simulink library "Bit_Multiplexers_Lib"  (R2023a)
settings: Solver=ode45  StartTime=0.0  StopTime=10.0  RelTol=1e-3  EnableMultiTasking=on
settings Model: Creator=uzivatel  LastModifiedBy=Jozko Mrkvicka
settings SolverCC: AlgebraicLoopSolver=TrustRegion
settings DataIOCC: LimitDataPoints=on  SaveFormat=Array  ReturnWorkspaceOutputs=off
settings OptimizationCC: LifeSpan=inf
settings DebuggingCC: UnderspecifiedInitializationDetection=Classic  MergeDetectMultiDrivingBlocksExec=none  SolverPrmCheckMsg=warning  UnconnectedInputMsg=warning  UnconnectedOutputMsg=warning  UnconnectedLineMsg=warning  StateNameClashWarn=warning  SFUnexpectedBacktrackingDiag=warning  SFNoUnconditionalDefaultTransitionDiag=warning  ArithmeticOperatorsInVariantConditions=warning
settings HardwareCC: ProdBitPerPointer=32  ProdBitPerSizeT=32  ProdBitPerPtrDiffT=32  ProdLargestAtomicFloat=None  ProdIntDivRoundTo=Undefined  ProdEndianess=Unspecified  ProdWordSize=32  ProdHWDeviceType=32-bit Generic
settings ModelReferenceCC: EnableRefExpFcnMdlSchedulingChecks=on  PropagateSignalLabelsOutOfModel=off
settings SFSimCC: SimUseLocalCustomCode=off  CustomCodeUndefinedFunction=UseInterfaceOnly
settings RTWCC: RTWUseLocalCustomCode=off
settings CodeAppCC: StateflowObjectComments=on
settings GRTTargetCC: TargetLangStandard=C89/C90 (ANSI)
settings ConfigComp: CovMetricSettings=dw  CovSaveCumulativeToWorkspaceVar=on  CovSaveSingleToWorkspaceVar=on  CovExternalEMLEnable=off

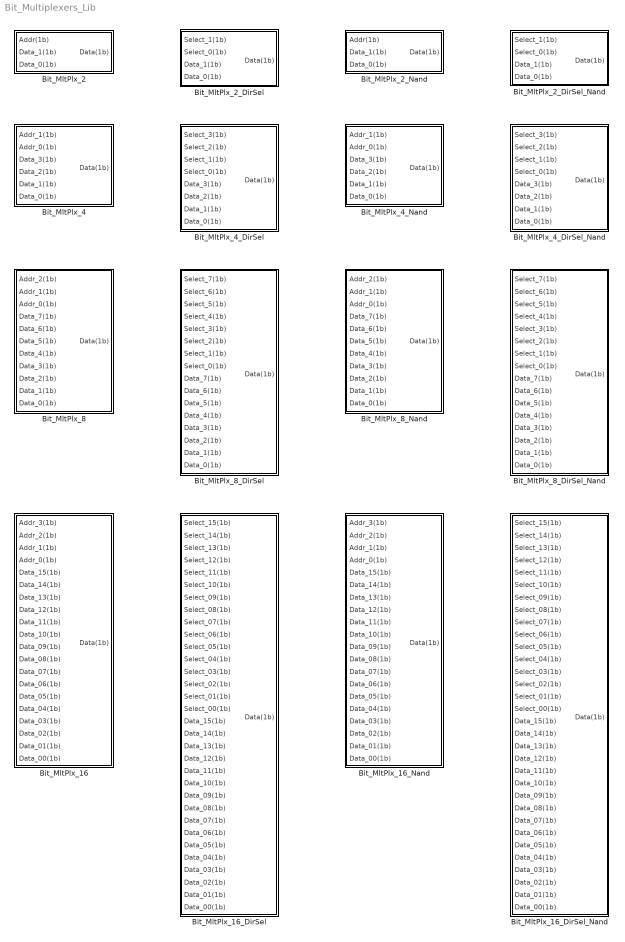
== system Bit_Multiplexers_Lib ==
  Bit_MltPlx_16 : Subsystem
  Bit_MltPlx_16_DirSel : Subsystem
  Bit_MltPlx_16_DirSel_Nand : Subsystem
  Bit_MltPlx_16_Nand : Subsystem
  Bit_MltPlx_2 : Subsystem
  Bit_MltPlx_2_DirSel : Subsystem
  Bit_MltPlx_2_DirSel_Nand : Subsystem
  Bit_MltPlx_2_Nand : Subsystem
  Bit_MltPlx_4 : Subsystem
  Bit_MltPlx_4_DirSel : Subsystem
  Bit_MltPlx_4_DirSel_Nand : Subsystem
  Bit_MltPlx_4_Nand : Subsystem
  Bit_MltPlx_8 : Subsystem
  Bit_MltPlx_8_DirSel : Subsystem
  Bit_MltPlx_8_DirSel_Nand : Subsystem
  Bit_MltPlx_8_Nand : Subsystem

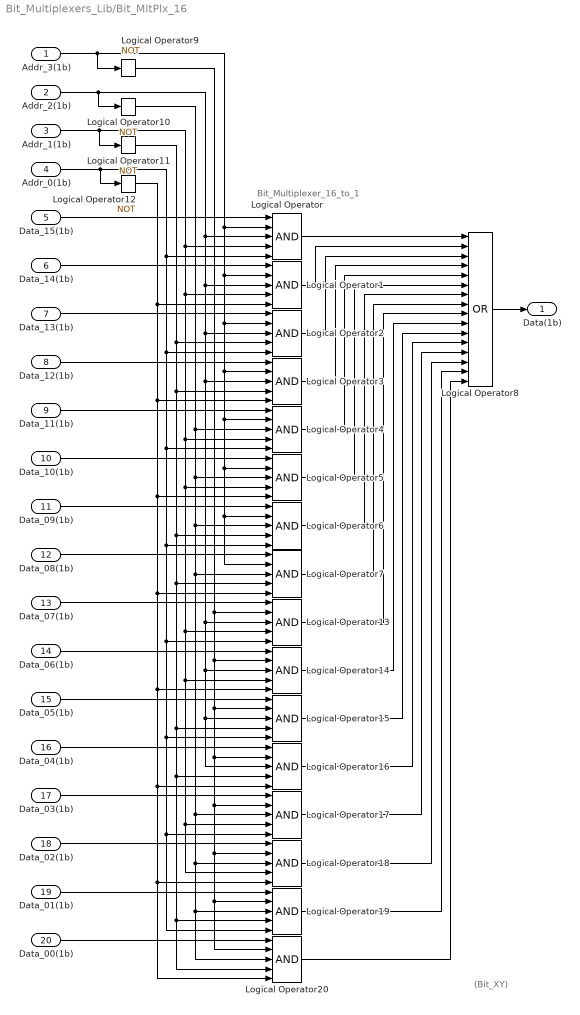
== system Bit_Multiplexers_Lib/Bit_MltPlx_16 ==
  note: (Bit_XY)
  note: Bit_Multiplexer_16_to_1
  Addr_3(1b) : Inport
  Addr_2(1b) : Inport  Port=2
  Addr_1(1b) : Inport  Port=3
  Addr_0(1b) : Inport  Port=4
  Data_15(1b) : Inport  Port=5
  Data_14(1b) : Inport  Port=6
  Data_13(1b) : Inport  Port=7
  Data_12(1b) : Inport  Port=8
  Data_11(1b) : Inport  Port=9
  Data_10(1b) : Inport  Port=10
  Data_09(1b) : Inport  Port=11
  Data_08(1b) : Inport  Port=12
  Data_07(1b) : Inport  Port=13
  Data_06(1b) : Inport  Port=14
  Data_05(1b) : Inport  Port=15
  Data_04(1b) : Inport  Port=16
  Data_03(1b) : Inport  Port=17
  Data_02(1b) : Inport  Port=18
  Data_01(1b) : Inport  Port=19
  Data_00(1b) : Inport  Port=20
  Logical Operator{,1..7,13..20} (16 alike) : Logic  Inputs=5  IconShape=distinctive  AllPortsSameDT=off  OutDataTypeStr=boolean
  Logical Operator{9..12} (4 alike) : Logic  Operator=NOT  Inputs=4  IconShape=distinctive  AllPortsSameDT=off  OutDataTypeStr=boolean
  Logical Operator8 : Logic  Operator=OR  Inputs=16  IconShape=distinctive  OutDataTypeStr=boolean
  Data(1b) : Outport
  wires:
  Logical Operator12/1 -> Logical Operator20/5, Logical Operator18/5, Logical Operator16/5, Logical Operator14/5, Logical Operator7/5, Logical Operator5/5, Logical Operator3/5, Logical Operator1/5
  Addr_0(1b)/1 -> Logical Operator19/5, Logical Operator17/5, Logical Operator15/5, Logical Operator13/5, Logical Operator6/5, Logical Operator4/5, Logical Operator2/5, Logical Operator/5, Logical Operator12/1
  Logical Operator11/1 -> Logical Operator20/4, Logical Operator19/4, Logical Operator16/4, Logical Operator15/4, Logical Operator7/4, Logical Operator6/4, Logical Operator3/4, Logical Operator2/4
  Addr_1(1b)/1 -> Logical Operator18/4, Logical Operator17/4, Logical Operator14/4, Logical Operator13/4, Logical Operator5/4, Logical Operator4/4, Logical Operator1/4, Logical Operator/4, Logical Operator11/1
  Logical Operator10/1 -> Logical Operator20/3, Logical Operator19/3, Logical Operator18/3, Logical Operator17/3, Logical Operator7/3, Logical Operator6/3, Logical Operator5/3, Logical Operator4/3
  Addr_2(1b)/1 -> Logical Operator16/3, Logical Operator15/3, Logical Operator14/3, Logical Operator13/3, Logical Operator3/3, Logical Operator2/3, Logical Operator1/3, Logical Operator/3, Logical Operator10/1
  Logical Operator9/1 -> Logical Operator20/2, Logical Operator19/2, Logical Operator18/2, Logical Operator17/2, Logical Operator16/2, Logical Operator15/2, Logical Operator14/2, Logical Operator13/2
  Addr_3(1b)/1 -> Logical Operator7/2, Logical Operator6/2, Logical Operator5/2, Logical Operator4/2, Logical Operator3/2, Logical Operator2/2, Logical Operator1/2, Logical Operator/2, Logical Operator9/1
  Data_00(1b)/1 -> Logical Operator20/1
  Data_01(1b)/1 -> Logical Operator19/1
  Data_02(1b)/1 -> Logical Operator18/1
  Data_03(1b)/1 -> Logical Operator17/1
  Data_04(1b)/1 -> Logical Operator16/1
  Data_05(1b)/1 -> Logical Operator15/1
  Data_06(1b)/1 -> Logical Operator14/1
  Data_07(1b)/1 -> Logical Operator13/1
  Logical Operator20/1 -> Logical Operator8/16
  Logical Operator19/1 -> Logical Operator8/15
  Logical Operator18/1 -> Logical Operator8/14
  Logical Operator17/1 -> Logical Operator8/13
  Logical Operator16/1 -> Logical Operator8/12
  Logical Operator15/1 -> Logical Operator8/11
  Logical Operator14/1 -> Logical Operator8/10
  Logical Operator13/1 -> Logical Operator8/9
  Logical Operator8/1 -> Data(1b)/1
  Data_15(1b)/1 -> Logical Operator/1
  Data_14(1b)/1 -> Logical Operator1/1
  Data_13(1b)/1 -> Logical Operator2/1
  Data_12(1b)/1 -> Logical Operator3/1
  Data_11(1b)/1 -> Logical Operator4/1
  Data_10(1b)/1 -> Logical Operator5/1
  Data_09(1b)/1 -> Logical Operator6/1
  Data_08(1b)/1 -> Logical Operator7/1
  Logical Operator7/1 -> Logical Operator8/8
  Logical Operator6/1 -> Logical Operator8/7
  Logical Operator5/1 -> Logical Operator8/6
  Logical Operator4/1 -> Logical Operator8/5
  Logical Operator3/1 -> Logical Operator8/4
  Logical Operator2/1 -> Logical Operator8/3
  Logical Operator1/1 -> Logical Operator8/2
  Logical Operator/1 -> Logical Operator8/1

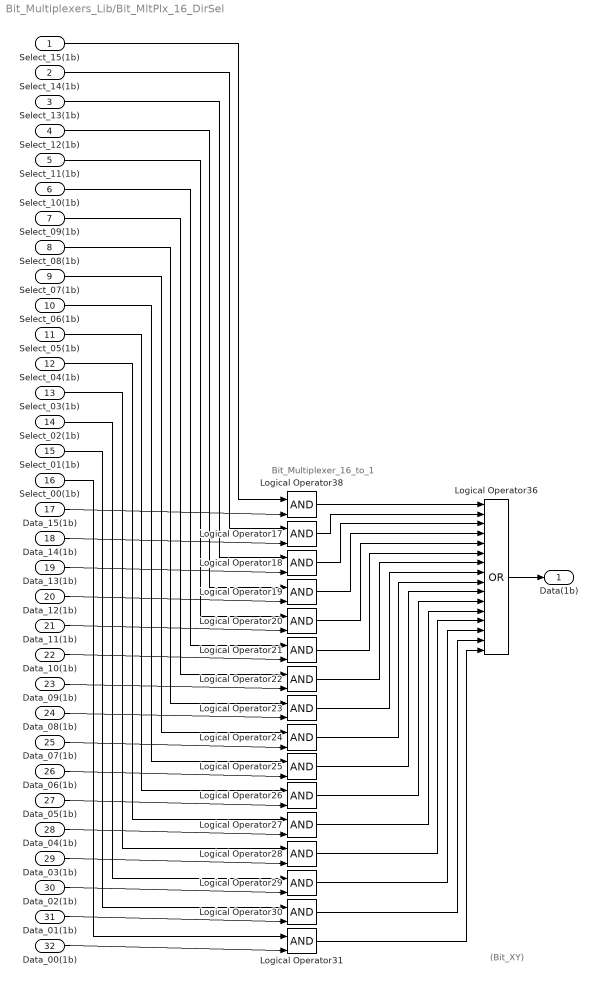
== system Bit_Multiplexers_Lib/Bit_MltPlx_16_DirSel ==
  note: Bit_Multiplexer_16_to_1
  note: (Bit_XY)
  Select_15(1b) : Inport
  Select_14(1b) : Inport  Port=2
  Select_13(1b) : Inport  Port=3
  Select_12(1b) : Inport  Port=4
  Select_11(1b) : Inport  Port=5
  Select_10(1b) : Inport  Port=6
  Select_09(1b) : Inport  Port=7
  Select_08(1b) : Inport  Port=8
  Select_07(1b) : Inport  Port=9
  Select_06(1b) : Inport  Port=10
  Select_05(1b) : Inport  Port=11
  Select_04(1b) : Inport  Port=12
  Select_03(1b) : Inport  Port=13
  Select_02(1b) : Inport  Port=14
  Select_01(1b) : Inport  Port=15
  Select_00(1b) : Inport  Port=16
  Data_15(1b) : Inport  Port=17
  Data_14(1b) : Inport  Port=18
  Data_13(1b) : Inport  Port=19
  Data_12(1b) : Inport  Port=20
  Data_11(1b) : Inport  Port=21
  Data_10(1b) : Inport  Port=22
  Data_09(1b) : Inport  Port=23
  Data_08(1b) : Inport  Port=24
  Data_07(1b) : Inport  Port=25
  Data_06(1b) : Inport  Port=26
  Data_05(1b) : Inport  Port=27
  Data_04(1b) : Inport  Port=28
  Data_03(1b) : Inport  Port=29
  Data_02(1b) : Inport  Port=30
  Data_01(1b) : Inport  Port=31
  Data_00(1b) : Inport  Port=32
  Logical Operator{17..31,38} (16 alike) : Logic  IconShape=distinctive  AllPortsSameDT=off  OutDataTypeStr=boolean
  Logical Operator36 : Logic  Operator=OR  Inputs=16  IconShape=distinctive  OutDataTypeStr=boolean
  Data(1b) : Outport
  wires:
  Data_03(1b)/1 -> Logical Operator28/2
  Logical Operator28/1 -> Logical Operator36/13
  Logical Operator36/1 -> Data(1b)/1
  Data_09(1b)/1 -> Logical Operator22/2
  Logical Operator20/1 -> Logical Operator36/5
  Data_14(1b)/1 -> Logical Operator17/2
  Logical Operator38/1 -> Logical Operator36/1
  Data_04(1b)/1 -> Logical Operator27/2
  Logical Operator19/1 -> Logical Operator36/4
  Data_08(1b)/1 -> Logical Operator23/2
  Logical Operator25/1 -> Logical Operator36/10
  Logical Operator27/1 -> Logical Operator36/12
  Logical Operator18/1 -> Logical Operator36/3
  Data_00(1b)/1 -> Logical Operator31/2
  Logical Operator17/1 -> Logical Operator36/2
  Data_05(1b)/1 -> Logical Operator26/2
  Logical Operator24/1 -> Logical Operator36/9
  Data_13(1b)/1 -> Logical Operator18/2
  Logical Operator30/1 -> Logical Operator36/15
  Logical Operator21/1 -> Logical Operator36/6
  Data_01(1b)/1 -> Logical Operator30/2
  Data_07(1b)/1 -> Logical Operator24/2
  Data_15(1b)/1 -> Logical Operator38/2
  Logical Operator31/1 -> Logical Operator36/16
  Data_06(1b)/1 -> Logical Operator25/2
  Data_11(1b)/1 -> Logical Operator20/2
  Logical Operator26/1 -> Logical Operator36/11
  Data_02(1b)/1 -> Logical Operator29/2
  Logical Operator22/1 -> Logical Operator36/7
  Logical Operator29/1 -> Logical Operator36/14
  Logical Operator23/1 -> Logical Operator36/8
  Data_10(1b)/1 -> Logical Operator21/2
  Data_12(1b)/1 -> Logical Operator19/2
  Select_06(1b)/1 -> Logical Operator25/1
  Select_03(1b)/1 -> Logical Operator28/1
  Select_10(1b)/1 -> Logical Operator21/1
  Select_02(1b)/1 -> Logical Operator29/1
  Select_07(1b)/1 -> Logical Operator24/1
  Select_05(1b)/1 -> Logical Operator26/1
  Select_04(1b)/1 -> Logical Operator27/1
  Select_09(1b)/1 -> Logical Operator22/1
  Select_14(1b)/1 -> Logical Operator17/1
  Select_13(1b)/1 -> Logical Operator18/1
  Select_11(1b)/1 -> Logical Operator20/1
  Select_01(1b)/1 -> Logical Operator30/1
  Select_15(1b)/1 -> Logical Operator38/1
  Select_00(1b)/1 -> Logical Operator31/1
  Select_08(1b)/1 -> Logical Operator23/1
  Select_12(1b)/1 -> Logical Operator19/1

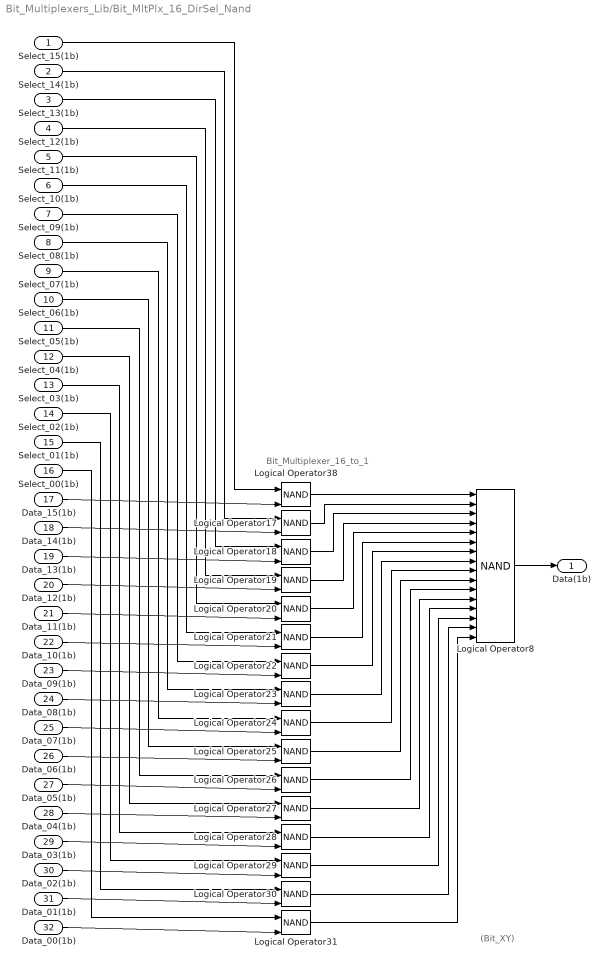
== system Bit_Multiplexers_Lib/Bit_MltPlx_16_DirSel_Nand ==
  note: Bit_Multiplexer_16_to_1
  note: (Bit_XY)
  Select_15(1b) : Inport
  Select_14(1b) : Inport  Port=2
  Select_13(1b) : Inport  Port=3
  Select_12(1b) : Inport  Port=4
  Select_11(1b) : Inport  Port=5
  Select_10(1b) : Inport  Port=6
  Select_09(1b) : Inport  Port=7
  Select_08(1b) : Inport  Port=8
  Select_07(1b) : Inport  Port=9
  Select_06(1b) : Inport  Port=10
  Select_05(1b) : Inport  Port=11
  Select_04(1b) : Inport  Port=12
  Select_03(1b) : Inport  Port=13
  Select_02(1b) : Inport  Port=14
  Select_01(1b) : Inport  Port=15
  Select_00(1b) : Inport  Port=16
  Data_15(1b) : Inport  Port=17
  Data_14(1b) : Inport  Port=18
  Data_13(1b) : Inport  Port=19
  Data_12(1b) : Inport  Port=20
  Data_11(1b) : Inport  Port=21
  Data_10(1b) : Inport  Port=22
  Data_09(1b) : Inport  Port=23
  Data_08(1b) : Inport  Port=24
  Data_07(1b) : Inport  Port=25
  Data_06(1b) : Inport  Port=26
  Data_05(1b) : Inport  Port=27
  Data_04(1b) : Inport  Port=28
  Data_03(1b) : Inport  Port=29
  Data_02(1b) : Inport  Port=30
  Data_01(1b) : Inport  Port=31
  Data_00(1b) : Inport  Port=32
  Logical Operator{17..31,38} (16 alike) : Logic  Operator=NAND  IconShape=distinctive  AllPortsSameDT=off  OutDataTypeStr=boolean
  Logical Operator8 : Logic  Operator=NAND  Inputs=16  IconShape=distinctive  OutDataTypeStr=boolean
  Data(1b) : Outport
  wires:
  Data_03(1b)/1 -> Logical Operator28/2
  Logical Operator28/1 -> Logical Operator8/13
  Logical Operator8/1 -> Data(1b)/1
  Data_09(1b)/1 -> Logical Operator22/2
  Logical Operator20/1 -> Logical Operator8/5
  Data_14(1b)/1 -> Logical Operator17/2
  Logical Operator38/1 -> Logical Operator8/1
  Data_04(1b)/1 -> Logical Operator27/2
  Logical Operator19/1 -> Logical Operator8/4
  Data_08(1b)/1 -> Logical Operator23/2
  Logical Operator25/1 -> Logical Operator8/10
  Logical Operator27/1 -> Logical Operator8/12
  Logical Operator18/1 -> Logical Operator8/3
  Data_00(1b)/1 -> Logical Operator31/2
  Logical Operator17/1 -> Logical Operator8/2
  Data_05(1b)/1 -> Logical Operator26/2
  Logical Operator24/1 -> Logical Operator8/9
  Data_13(1b)/1 -> Logical Operator18/2
  Logical Operator30/1 -> Logical Operator8/15
  Logical Operator21/1 -> Logical Operator8/6
  Data_01(1b)/1 -> Logical Operator30/2
  Data_07(1b)/1 -> Logical Operator24/2
  Data_15(1b)/1 -> Logical Operator38/2
  Logical Operator31/1 -> Logical Operator8/16
  Data_06(1b)/1 -> Logical Operator25/2
  Data_11(1b)/1 -> Logical Operator20/2
  Logical Operator26/1 -> Logical Operator8/11
  Data_02(1b)/1 -> Logical Operator29/2
  Logical Operator22/1 -> Logical Operator8/7
  Logical Operator29/1 -> Logical Operator8/14
  Logical Operator23/1 -> Logical Operator8/8
  Data_10(1b)/1 -> Logical Operator21/2
  Data_12(1b)/1 -> Logical Operator19/2
  Select_06(1b)/1 -> Logical Operator25/1
  Select_03(1b)/1 -> Logical Operator28/1
  Select_10(1b)/1 -> Logical Operator21/1
  Select_02(1b)/1 -> Logical Operator29/1
  Select_07(1b)/1 -> Logical Operator24/1
  Select_05(1b)/1 -> Logical Operator26/1
  Select_04(1b)/1 -> Logical Operator27/1
  Select_09(1b)/1 -> Logical Operator22/1
  Select_14(1b)/1 -> Logical Operator17/1
  Select_13(1b)/1 -> Logical Operator18/1
  Select_11(1b)/1 -> Logical Operator20/1
  Select_01(1b)/1 -> Logical Operator30/1
  Select_15(1b)/1 -> Logical Operator38/1
  Select_00(1b)/1 -> Logical Operator31/1
  Select_08(1b)/1 -> Logical Operator23/1
  Select_12(1b)/1 -> Logical Operator19/1

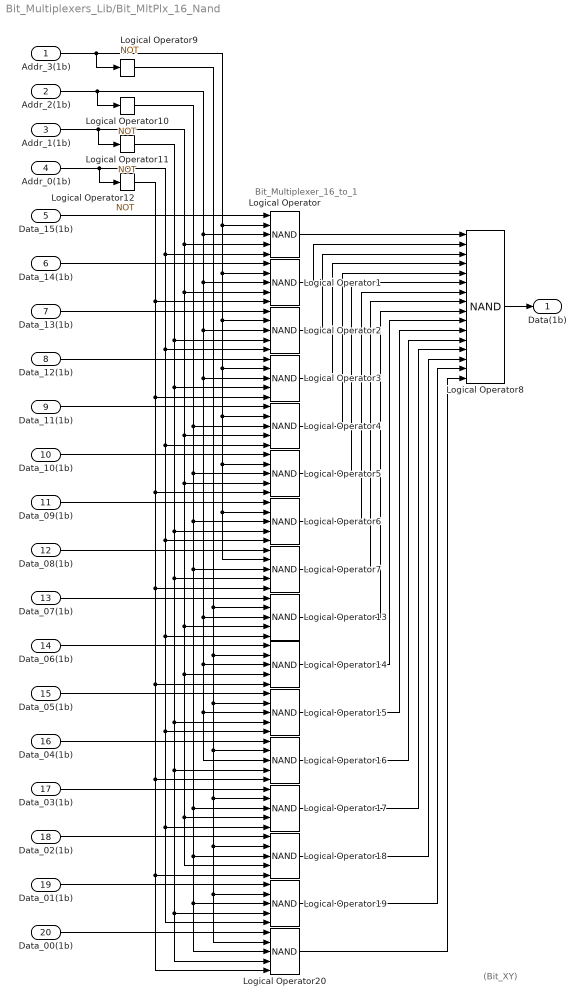
== system Bit_Multiplexers_Lib/Bit_MltPlx_16_Nand ==
  note: Bit_Multiplexer_16_to_1
  note: (Bit_XY)
  Addr_3(1b) : Inport
  Addr_2(1b) : Inport  Port=2
  Addr_1(1b) : Inport  Port=3
  Addr_0(1b) : Inport  Port=4
  Data_15(1b) : Inport  Port=5
  Data_14(1b) : Inport  Port=6
  Data_13(1b) : Inport  Port=7
  Data_12(1b) : Inport  Port=8
  Data_11(1b) : Inport  Port=9
  Data_10(1b) : Inport  Port=10
  Data_09(1b) : Inport  Port=11
  Data_08(1b) : Inport  Port=12
  Data_07(1b) : Inport  Port=13
  Data_06(1b) : Inport  Port=14
  Data_05(1b) : Inport  Port=15
  Data_04(1b) : Inport  Port=16
  Data_03(1b) : Inport  Port=17
  Data_02(1b) : Inport  Port=18
  Data_01(1b) : Inport  Port=19
  Data_00(1b) : Inport  Port=20
  Logical Operator{,1..7,13..20} (16 alike) : Logic  Operator=NAND  Inputs=5  IconShape=distinctive  AllPortsSameDT=off  OutDataTypeStr=boolean
  Logical Operator{9..12} (4 alike) : Logic  Operator=NOT  Inputs=4  IconShape=distinctive  AllPortsSameDT=off  OutDataTypeStr=boolean
  Logical Operator8 : Logic  Operator=NAND  Inputs=16  IconShape=distinctive  OutDataTypeStr=boolean
  Data(1b) : Outport
  wires:
  Data_03(1b)/1 -> Logical Operator17/1
  Logical Operator17/1 -> Logical Operator8/13
  Logical Operator8/1 -> Data(1b)/1
  Data_09(1b)/1 -> Logical Operator6/1
  Logical Operator9/1 -> Logical Operator20/2, Logical Operator19/2, Logical Operator18/2, Logical Operator17/2, Logical Operator16/2, Logical Operator15/2, Logical Operator14/2, Logical Operator13/2
  Addr_2(1b)/1 -> Logical Operator16/3, Logical Operator15/3, Logical Operator14/3, Logical Operator13/3, Logical Operator3/3, Logical Operator2/3, Logical Operator1/3, Logical Operator/3, Logical Operator10/1
  Logical Operator11/1 -> Logical Operator20/4, Logical Operator19/4, Logical Operator16/4, Logical Operator15/4, Logical Operator7/4, Logical Operator6/4, Logical Operator3/4, Logical Operator2/4
  Logical Operator12/1 -> Logical Operator20/5, Logical Operator18/5, Logical Operator16/5, Logical Operator14/5, Logical Operator7/5, Logical Operator5/5, Logical Operator3/5, Logical Operator1/5
  Logical Operator4/1 -> Logical Operator8/5
  Data_14(1b)/1 -> Logical Operator1/1
  Logical Operator/1 -> Logical Operator8/1
  Data_04(1b)/1 -> Logical Operator16/1
  Logical Operator3/1 -> Logical Operator8/4
  Addr_0(1b)/1 -> Logical Operator19/5, Logical Operator17/5, Logical Operator15/5, Logical Operator13/5, Logical Operator6/5, Logical Operator4/5, Logical Operator2/5, Logical Operator/5, Logical Operator12/1
  Data_08(1b)/1 -> Logical Operator7/1
  Logical Operator10/1 -> Logical Operator20/3, Logical Operator19/3, Logical Operator18/3, Logical Operator17/3, Logical Operator7/3, Logical Operator6/3, Logical Operator5/3, Logical Operator4/3
  Logical Operator14/1 -> Logical Operator8/10
  Logical Operator16/1 -> Logical Operator8/12
  Logical Operator2/1 -> Logical Operator8/3
  Addr_3(1b)/1 -> Logical Operator7/2, Logical Operator6/2, Logical Operator5/2, Logical Operator4/2, Logical Operator3/2, Logical Operator2/2, Logical Operator1/2, Logical Operator/2, Logical Operator9/1
  Data_00(1b)/1 -> Logical Operator20/1
  Logical Operator1/1 -> Logical Operator8/2
  Data_05(1b)/1 -> Logical Operator15/1
  Logical Operator13/1 -> Logical Operator8/9
  Data_13(1b)/1 -> Logical Operator2/1
  Logical Operator19/1 -> Logical Operator8/15
  Logical Operator5/1 -> Logical Operator8/6
  Data_01(1b)/1 -> Logical Operator19/1
  Data_07(1b)/1 -> Logical Operator13/1
  Data_15(1b)/1 -> Logical Operator/1
  Logical Operator20/1 -> Logical Operator8/16
  Data_06(1b)/1 -> Logical Operator14/1
  Data_11(1b)/1 -> Logical Operator4/1
  Addr_1(1b)/1 -> Logical Operator18/4, Logical Operator17/4, Logical Operator14/4, Logical Operator13/4, Logical Operator5/4, Logical Operator4/4, Logical Operator1/4, Logical Operator/4, Logical Operator11/1
  Logical Operator15/1 -> Logical Operator8/11
  Data_02(1b)/1 -> Logical Operator18/1
  Logical Operator6/1 -> Logical Operator8/7
  Logical Operator18/1 -> Logical Operator8/14
  Logical Operator7/1 -> Logical Operator8/8
  Data_10(1b)/1 -> Logical Operator5/1
  Data_12(1b)/1 -> Logical Operator3/1

== system Bit_Multiplexers_Lib/Bit_MltPlx_2 ==
  note: ( Bit_XY )
  note: Bit_Multiplexer_2_to_1
  Addr(1b) : Inport
  Data_1(1b) : Inport  Port=2
  Data_0(1b) : Inport  Port=3
  Logical Operator1 : Logic  IconShape=distinctive  AllPortsSameDT=off  OutDataTypeStr=boolean
  Logical Operator12 : Logic  Operator=NOT  Inputs=4  IconShape=distinctive  AllPortsSameDT=off  OutDataTypeStr=boolean
  Logical Operator21 : Logic  IconShape=distinctive  AllPortsSameDT=off  OutDataTypeStr=boolean
  Logical Operator64 : Logic  Operator=OR  IconShape=distinctive  OutDataTypeStr=boolean
  Data(1b) : Outport
  wires:
  Logical Operator12/1 -> Logical Operator21/1
  Addr(1b)/1 -> Logical Operator1/1, Logical Operator12/1
  Data_0(1b)/1 -> Logical Operator21/2
  Data_1(1b)/1 -> Logical Operator1/2
  Logical Operator64/1 -> Data(1b)/1
  Logical Operator1/1 -> Logical Operator64/1
  Logical Operator21/1 -> Logical Operator64/2

== system Bit_Multiplexers_Lib/Bit_MltPlx_2_DirSel ==
  note: ( Bit_XY )
  note: Bit_Multiplexer_2_to_1
  Select_1(1b) : Inport
  Select_0(1b) : Inport  Port=2
  Data_1(1b) : Inport  Port=3
  Data_0(1b) : Inport  Port=4
  Logical Operator1 : Logic  IconShape=distinctive  AllPortsSameDT=off  OutDataTypeStr=boolean
  Logical Operator21 : Logic  IconShape=distinctive  AllPortsSameDT=off  OutDataTypeStr=boolean
  Logical Operator64 : Logic  Operator=OR  IconShape=distinctive  OutDataTypeStr=boolean
  Data(1b) : Outport
  wires:
  Select_1(1b)/1 -> Logical Operator1/1
  Select_0(1b)/1 -> Logical Operator21/1
  Data_0(1b)/1 -> Logical Operator21/2
  Data_1(1b)/1 -> Logical Operator1/2
  Logical Operator1/1 -> Logical Operator64/1
  Logical Operator64/1 -> Data(1b)/1
  Logical Operator21/1 -> Logical Operator64/2

== system Bit_Multiplexers_Lib/Bit_MltPlx_2_DirSel_Nand ==
  note: Bit_Multiplexer_2_to_1
  note: ( Bit_XY )
  Select_1(1b) : Inport
  Select_0(1b) : Inport  Port=2
  Data_1(1b) : Inport  Port=3
  Data_0(1b) : Inport  Port=4
  Logical Operator1 : Logic  Operator=NAND  IconShape=distinctive  AllPortsSameDT=off  OutDataTypeStr=boolean
  Logical Operator21 : Logic  Operator=NAND  IconShape=distinctive  AllPortsSameDT=off  OutDataTypeStr=boolean
  Logical Operator64 : Logic  Operator=NAND  IconShape=distinctive  OutDataTypeStr=boolean
  Data(1b) : Outport
  wires:
  Data_1(1b)/1 -> Logical Operator1/2
  Select_0(1b)/1 -> Logical Operator21/1
  Data_0(1b)/1 -> Logical Operator21/2
  Select_1(1b)/1 -> Logical Operator1/1
  Logical Operator64/1 -> Data(1b)/1
  Logical Operator21/1 -> Logical Operator64/2
  Logical Operator1/1 -> Logical Operator64/1

== system Bit_Multiplexers_Lib/Bit_MltPlx_2_Nand ==
  note: Bit_Multiplexer_2_to_1
  note: ( Bit_XY )
  Addr(1b) : Inport
  Data_1(1b) : Inport  Port=2
  Data_0(1b) : Inport  Port=3
  Logical Operator12 : Logic  Operator=NOT  Inputs=4  IconShape=distinctive  AllPortsSameDT=off  OutDataTypeStr=boolean
  Logical Operator2 : Logic  Operator=NAND  IconShape=distinctive  AllPortsSameDT=off  OutDataTypeStr=boolean
  Logical Operator21 : Logic  Operator=NAND  IconShape=distinctive  AllPortsSameDT=off  OutDataTypeStr=boolean
  Logical Operator64 : Logic  Operator=NAND  IconShape=distinctive  OutDataTypeStr=boolean
  Data(1b) : Outport
  wires:
  Data_0(1b)/1 -> Logical Operator21/2
  Logical Operator12/1 -> Logical Operator21/1
  Addr(1b)/1 -> Logical Operator2/1, Logical Operator12/1
  Data_1(1b)/1 -> Logical Operator2/2
  Logical Operator21/1 -> Logical Operator64/2
  Logical Operator2/1 -> Logical Operator64/1
  Logical Operator64/1 -> Data(1b)/1

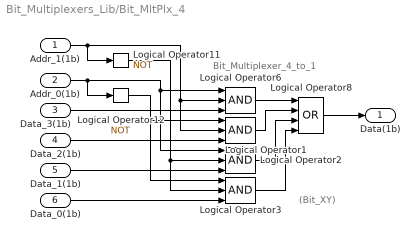
== system Bit_Multiplexers_Lib/Bit_MltPlx_4 ==
  note: Bit_Multiplexer_4_to_1
  note: (Bit_XY)
  Addr_1(1b) : Inport
  Addr_0(1b) : Inport  Port=2
  Data_3(1b) : Inport  Port=3
  Data_2(1b) : Inport  Port=4
  Data_1(1b) : Inport  Port=5
  Data_0(1b) : Inport  Port=6
  Logical Operator{1..3,6} (4 alike) : Logic  Inputs=3  IconShape=distinctive  AllPortsSameDT=off  OutDataTypeStr=boolean
  Logical Operator11 : Logic  Operator=NOT  Inputs=4  IconShape=distinctive  AllPortsSameDT=off  OutDataTypeStr=boolean
  Logical Operator12 : Logic  Operator=NOT  Inputs=4  IconShape=distinctive  AllPortsSameDT=off  OutDataTypeStr=boolean
  Logical Operator8 : Logic  Operator=OR  Inputs=4  IconShape=distinctive  OutDataTypeStr=boolean
  Data(1b) : Outport
  wires:
  Logical Operator12/1 -> Logical Operator3/1, Logical Operator1/1
  Addr_0(1b)/1 -> Logical Operator2/1, Logical Operator6/1, Logical Operator12/1
  Logical Operator11/1 -> Logical Operator3/2, Logical Operator2/2
  Addr_1(1b)/1 -> Logical Operator1/2, Logical Operator6/2, Logical Operator11/1
  Data_3(1b)/1 -> Logical Operator6/3
  Data_2(1b)/1 -> Logical Operator1/3
  Data_1(1b)/1 -> Logical Operator2/3
  Data_0(1b)/1 -> Logical Operator3/3
  Logical Operator6/1 -> Logical Operator8/1
  Logical Operator1/1 -> Logical Operator8/2
  Logical Operator8/1 -> Data(1b)/1
  Logical Operator2/1 -> Logical Operator8/3
  Logical Operator3/1 -> Logical Operator8/4

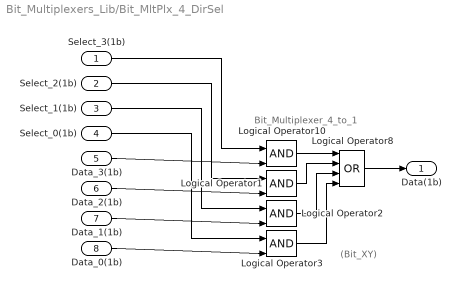
== system Bit_Multiplexers_Lib/Bit_MltPlx_4_DirSel ==
  note: Bit_Multiplexer_4_to_1
  note: (Bit_XY)
  Select_3(1b) : Inport
  Select_2(1b) : Inport  Port=2
  Select_1(1b) : Inport  Port=3
  Select_0(1b) : Inport  Port=4
  Data_3(1b) : Inport  Port=5
  Data_2(1b) : Inport  Port=6
  Data_1(1b) : Inport  Port=7
  Data_0(1b) : Inport  Port=8
  Logical Operator{1..3,10} (4 alike) : Logic  IconShape=distinctive  AllPortsSameDT=off  OutDataTypeStr=boolean
  Logical Operator8 : Logic  Operator=OR  Inputs=4  IconShape=distinctive  OutDataTypeStr=boolean
  Data(1b) : Outport
  wires:
  Data_3(1b)/1 -> Logical Operator10/2
  Data_2(1b)/1 -> Logical Operator1/2
  Data_1(1b)/1 -> Logical Operator2/2
  Data_0(1b)/1 -> Logical Operator3/2
  Select_3(1b)/1 -> Logical Operator10/1
  Select_2(1b)/1 -> Logical Operator1/1
  Select_1(1b)/1 -> Logical Operator2/1
  Select_0(1b)/1 -> Logical Operator3/1
  Logical Operator10/1 -> Logical Operator8/1
  Logical Operator2/1 -> Logical Operator8/3
  Logical Operator3/1 -> Logical Operator8/4
  Logical Operator1/1 -> Logical Operator8/2
  Logical Operator8/1 -> Data(1b)/1

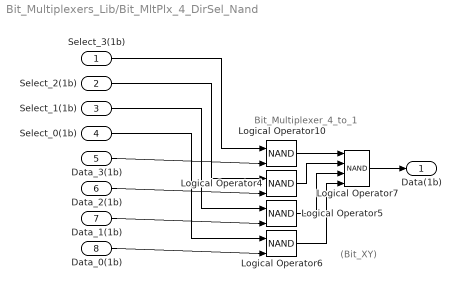
== system Bit_Multiplexers_Lib/Bit_MltPlx_4_DirSel_Nand ==
  note: (Bit_XY)
  note: Bit_Multiplexer_4_to_1
  Select_3(1b) : Inport
  Select_2(1b) : Inport  Port=2
  Select_1(1b) : Inport  Port=3
  Select_0(1b) : Inport  Port=4
  Data_3(1b) : Inport  Port=5
  Data_2(1b) : Inport  Port=6
  Data_1(1b) : Inport  Port=7
  Data_0(1b) : Inport  Port=8
  Logical Operator{4..6,10} (4 alike) : Logic  Operator=NAND  IconShape=distinctive  AllPortsSameDT=off  OutDataTypeStr=boolean
  Logical Operator7 : Logic  Operator=NAND  Inputs=4  IconShape=distinctive  OutDataTypeStr=boolean
  Data(1b) : Outport
  wires:
  Select_2(1b)/1 -> Logical Operator4/1
  Data_2(1b)/1 -> Logical Operator4/2
  Select_1(1b)/1 -> Logical Operator5/1
  Select_3(1b)/1 -> Logical Operator10/1
  Data_0(1b)/1 -> Logical Operator6/2
  Data_3(1b)/1 -> Logical Operator10/2
  Select_0(1b)/1 -> Logical Operator6/1
  Data_1(1b)/1 -> Logical Operator5/2
  Logical Operator4/1 -> Logical Operator7/2
  Logical Operator6/1 -> Logical Operator7/4
  Logical Operator5/1 -> Logical Operator7/3
  Logical Operator7/1 -> Data(1b)/1
  Logical Operator10/1 -> Logical Operator7/1

== system Bit_Multiplexers_Lib/Bit_MltPlx_4_Nand ==
  note: Bit_Multiplexer_4_to_1
  note: (Bit_XY)
  Addr_1(1b) : Inport
  Addr_0(1b) : Inport  Port=2
  Data_3(1b) : Inport  Port=3
  Data_2(1b) : Inport  Port=4
  Data_1(1b) : Inport  Port=5
  Data_0(1b) : Inport  Port=6
  Logical Operator{4,7,9..10} (4 alike) : Logic  Operator=NAND  Inputs=3  IconShape=distinctive  AllPortsSameDT=off  OutDataTypeStr=boolean
  Logical Operator13 : Logic  Operator=NAND  Inputs=4  IconShape=distinctive  OutDataTypeStr=boolean
  Logical Operator5 : Logic  Operator=NOT  Inputs=4  IconShape=distinctive  AllPortsSameDT=off  OutDataTypeStr=boolean
  Logical Operator6 : Logic  Operator=NOT  Inputs=4  IconShape=distinctive  AllPortsSameDT=off  OutDataTypeStr=boolean
  Data(1b) : Outport
  wires:
  Data_1(1b)/1 -> Logical Operator7/3
  Data_0(1b)/1 -> Logical Operator9/3
  Data_2(1b)/1 -> Logical Operator4/3
  Addr_0(1b)/1 -> Logical Operator10/1, Logical Operator7/1, Logical Operator6/1
  Logical Operator5/1 -> Logical Operator7/2, Logical Operator9/2
  Logical Operator6/1 -> Logical Operator4/1, Logical Operator9/1
  Addr_1(1b)/1 -> Logical Operator10/2, Logical Operator4/2, Logical Operator5/1
  Data_3(1b)/1 -> Logical Operator10/3
  Logical Operator4/1 -> Logical Operator13/2
  Logical Operator7/1 -> Logical Operator13/3
  Logical Operator13/1 -> Data(1b)/1
  Logical Operator9/1 -> Logical Operator13/4
  Logical Operator10/1 -> Logical Operator13/1

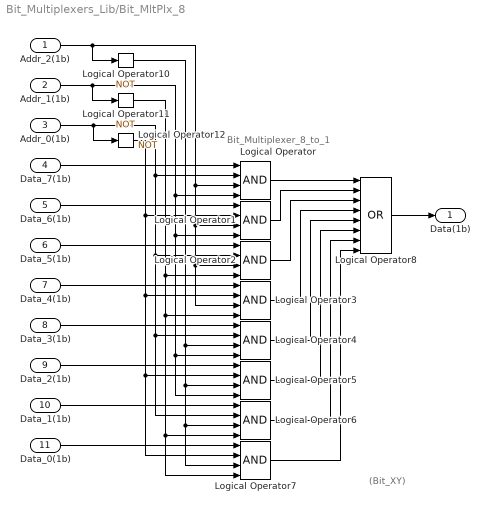
== system Bit_Multiplexers_Lib/Bit_MltPlx_8 ==
  note: (Bit_XY)
  note: Bit_Multiplexer_8_to_1
  Addr_2(1b) : Inport
  Addr_1(1b) : Inport  Port=2
  Addr_0(1b) : Inport  Port=3
  Data_7(1b) : Inport  Port=4
  Data_6(1b) : Inport  Port=5
  Data_5(1b) : Inport  Port=6
  Data_4(1b) : Inport  Port=7
  Data_3(1b) : Inport  Port=8
  Data_2(1b) : Inport  Port=9
  Data_1(1b) : Inport  Port=10
  Data_0(1b) : Inport  Port=11
  Logical Operator{,1..7} (8 alike) : Logic  Inputs=4  IconShape=distinctive  AllPortsSameDT=off  OutDataTypeStr=boolean
  Logical Operator10 : Logic  Operator=NOT  Inputs=4  IconShape=distinctive  AllPortsSameDT=off  OutDataTypeStr=boolean
  Logical Operator11 : Logic  Operator=NOT  Inputs=4  IconShape=distinctive  AllPortsSameDT=off  OutDataTypeStr=boolean
  Logical Operator12 : Logic  Operator=NOT  Inputs=4  IconShape=distinctive  AllPortsSameDT=off  OutDataTypeStr=boolean
  Logical Operator8 : Logic  Operator=OR  Inputs=8  IconShape=distinctive  OutDataTypeStr=boolean
  Data(1b) : Outport
  wires:
  Logical Operator12/1 -> Logical Operator1/2, Logical Operator3/2, Logical Operator7/2, Logical Operator5/2
  Addr_0(1b)/1 -> Logical Operator12/1, Logical Operator/2, Logical Operator2/2, Logical Operator6/2, Logical Operator4/2
  Logical Operator11/1 -> Logical Operator2/4, Logical Operator3/4, Logical Operator7/4, Logical Operator6/4
  Addr_1(1b)/1 -> Logical Operator11/1, Logical Operator/4, Logical Operator1/4, Logical Operator5/4, Logical Operator4/4
  Logical Operator10/1 -> Logical Operator4/3, Logical Operator5/3, Logical Operator7/3, Logical Operator6/3
  Addr_2(1b)/1 -> Logical Operator/3, Logical Operator1/3, Logical Operator3/3, Logical Operator2/3, Logical Operator10/1
  Data_7(1b)/1 -> Logical Operator/1
  Data_6(1b)/1 -> Logical Operator1/1
  Data_5(1b)/1 -> Logical Operator2/1
  Data_4(1b)/1 -> Logical Operator3/1
  Data_3(1b)/1 -> Logical Operator4/1
  Data_2(1b)/1 -> Logical Operator5/1
  Data_1(1b)/1 -> Logical Operator6/1
  Data_0(1b)/1 -> Logical Operator7/1
  Logical Operator2/1 -> Logical Operator8/3
  Logical Operator3/1 -> Logical Operator8/4
  Logical Operator6/1 -> Logical Operator8/7
  Logical Operator/1 -> Logical Operator8/1
  Logical Operator5/1 -> Logical Operator8/6
  Logical Operator8/1 -> Data(1b)/1
  Logical Operator7/1 -> Logical Operator8/8
  Logical Operator1/1 -> Logical Operator8/2
  Logical Operator4/1 -> Logical Operator8/5

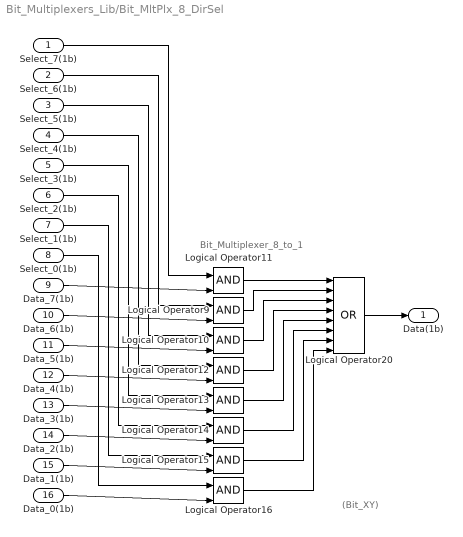
== system Bit_Multiplexers_Lib/Bit_MltPlx_8_DirSel ==
  note: (Bit_XY)
  note: Bit_Multiplexer_8_to_1
  Select_7(1b) : Inport
  Select_6(1b) : Inport  Port=2
  Select_5(1b) : Inport  Port=3
  Select_4(1b) : Inport  Port=4
  Select_3(1b) : Inport  Port=5
  Select_2(1b) : Inport  Port=6
  Select_1(1b) : Inport  Port=7
  Select_0(1b) : Inport  Port=8
  Data_7(1b) : Inport  Port=9
  Data_6(1b) : Inport  Port=10
  Data_5(1b) : Inport  Port=11
  Data_4(1b) : Inport  Port=12
  Data_3(1b) : Inport  Port=13
  Data_2(1b) : Inport  Port=14
  Data_1(1b) : Inport  Port=15
  Data_0(1b) : Inport  Port=16
  Logical Operator{9..16} (8 alike) : Logic  IconShape=distinctive  AllPortsSameDT=off  OutDataTypeStr=boolean
  Logical Operator20 : Logic  Operator=OR  Inputs=8  IconShape=distinctive  OutDataTypeStr=boolean
  Data(1b) : Outport
  wires:
  Data_3(1b)/1 -> Logical Operator13/2
  Data_4(1b)/1 -> Logical Operator12/2
  Logical Operator11/1 -> Logical Operator20/1
  Logical Operator10/1 -> Logical Operator20/3
  Logical Operator15/1 -> Logical Operator20/7
  Logical Operator9/1 -> Logical Operator20/2
  Logical Operator16/1 -> Logical Operator20/8
  Data_5(1b)/1 -> Logical Operator10/2
  Logical Operator20/1 -> Data(1b)/1
  Data_6(1b)/1 -> Logical Operator9/2
  Logical Operator12/1 -> Logical Operator20/4
  Data_7(1b)/1 -> Logical Operator11/2
  Logical Operator13/1 -> Logical Operator20/5
  Data_2(1b)/1 -> Logical Operator14/2
  Logical Operator14/1 -> Logical Operator20/6
  Data_0(1b)/1 -> Logical Operator16/2
  Data_1(1b)/1 -> Logical Operator15/2
  Select_0(1b)/1 -> Logical Operator16/1
  Select_3(1b)/1 -> Logical Operator13/1
  Select_2(1b)/1 -> Logical Operator14/1
  Select_1(1b)/1 -> Logical Operator15/1
  Select_4(1b)/1 -> Logical Operator12/1
  Select_6(1b)/1 -> Logical Operator9/1
  Select_7(1b)/1 -> Logical Operator11/1
  Select_5(1b)/1 -> Logical Operator10/1

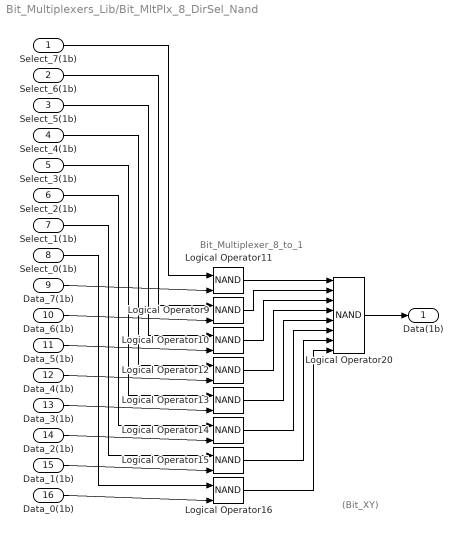
== system Bit_Multiplexers_Lib/Bit_MltPlx_8_DirSel_Nand ==
  note: (Bit_XY)
  note: Bit_Multiplexer_8_to_1
  Select_7(1b) : Inport
  Select_6(1b) : Inport  Port=2
  Select_5(1b) : Inport  Port=3
  Select_4(1b) : Inport  Port=4
  Select_3(1b) : Inport  Port=5
  Select_2(1b) : Inport  Port=6
  Select_1(1b) : Inport  Port=7
  Select_0(1b) : Inport  Port=8
  Data_7(1b) : Inport  Port=9
  Data_6(1b) : Inport  Port=10
  Data_5(1b) : Inport  Port=11
  Data_4(1b) : Inport  Port=12
  Data_3(1b) : Inport  Port=13
  Data_2(1b) : Inport  Port=14
  Data_1(1b) : Inport  Port=15
  Data_0(1b) : Inport  Port=16
  Logical Operator{9..16} (8 alike) : Logic  Operator=NAND  IconShape=distinctive  AllPortsSameDT=off  OutDataTypeStr=boolean
  Logical Operator20 : Logic  Operator=NAND  Inputs=8  IconShape=distinctive  OutDataTypeStr=boolean
  Data(1b) : Outport
  wires:
  Data_3(1b)/1 -> Logical Operator13/2
  Data_4(1b)/1 -> Logical Operator12/2
  Logical Operator11/1 -> Logical Operator20/1
  Logical Operator10/1 -> Logical Operator20/3
  Logical Operator15/1 -> Logical Operator20/7
  Logical Operator9/1 -> Logical Operator20/2
  Logical Operator16/1 -> Logical Operator20/8
  Data_5(1b)/1 -> Logical Operator10/2
  Logical Operator20/1 -> Data(1b)/1
  Data_6(1b)/1 -> Logical Operator9/2
  Logical Operator12/1 -> Logical Operator20/4
  Data_7(1b)/1 -> Logical Operator11/2
  Logical Operator13/1 -> Logical Operator20/5
  Data_2(1b)/1 -> Logical Operator14/2
  Logical Operator14/1 -> Logical Operator20/6
  Data_0(1b)/1 -> Logical Operator16/2
  Data_1(1b)/1 -> Logical Operator15/2
  Select_0(1b)/1 -> Logical Operator16/1
  Select_3(1b)/1 -> Logical Operator13/1
  Select_2(1b)/1 -> Logical Operator14/1
  Select_1(1b)/1 -> Logical Operator15/1
  Select_4(1b)/1 -> Logical Operator12/1
  Select_6(1b)/1 -> Logical Operator9/1
  Select_7(1b)/1 -> Logical Operator11/1
  Select_5(1b)/1 -> Logical Operator10/1

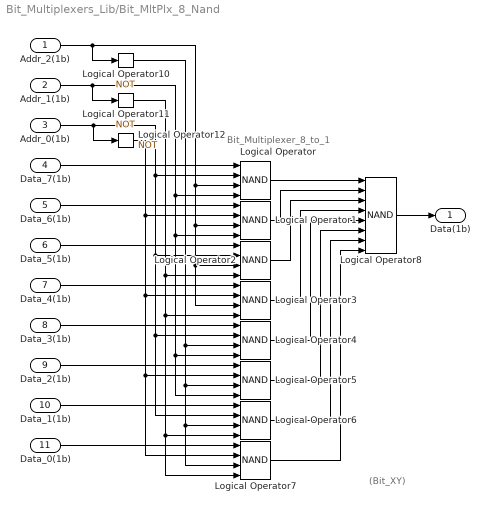
== system Bit_Multiplexers_Lib/Bit_MltPlx_8_Nand ==
  note: (Bit_XY)
  note: Bit_Multiplexer_8_to_1
  Addr_2(1b) : Inport
  Addr_1(1b) : Inport  Port=2
  Addr_0(1b) : Inport  Port=3
  Data_7(1b) : Inport  Port=4
  Data_6(1b) : Inport  Port=5
  Data_5(1b) : Inport  Port=6
  Data_4(1b) : Inport  Port=7
  Data_3(1b) : Inport  Port=8
  Data_2(1b) : Inport  Port=9
  Data_1(1b) : Inport  Port=10
  Data_0(1b) : Inport  Port=11
  Logical Operator{,1..7} (8 alike) : Logic  Operator=NAND  Inputs=4  IconShape=distinctive  AllPortsSameDT=off  OutDataTypeStr=boolean
  Logical Operator10 : Logic  Operator=NOT  Inputs=4  IconShape=distinctive  AllPortsSameDT=off  OutDataTypeStr=boolean
  Logical Operator11 : Logic  Operator=NOT  Inputs=4  IconShape=distinctive  AllPortsSameDT=off  OutDataTypeStr=boolean
  Logical Operator12 : Logic  Operator=NOT  Inputs=4  IconShape=distinctive  AllPortsSameDT=off  OutDataTypeStr=boolean
  Logical Operator8 : Logic  Operator=NAND  Inputs=8  IconShape=distinctive  OutDataTypeStr=boolean
  Data(1b) : Outport
  wires:
  Data_3(1b)/1 -> Logical Operator4/1
  Data_4(1b)/1 -> Logical Operator3/1
  Logical Operator12/1 -> Logical Operator1/2, Logical Operator3/2, Logical Operator7/2, Logical Operator5/2
  Logical Operator11/1 -> Logical Operator2/4, Logical Operator3/4, Logical Operator7/4, Logical Operator6/4
  Addr_1(1b)/1 -> Logical Operator11/1, Logical Operator/4, Logical Operator1/4, Logical Operator5/4, Logical Operator4/4
  Addr_0(1b)/1 -> Logical Operator12/1, Logical Operator/2, Logical Operator2/2, Logical Operator6/2, Logical Operator4/2
  Logical Operator/1 -> Logical Operator8/1
  Logical Operator2/1 -> Logical Operator8/3
  Logical Operator6/1 -> Logical Operator8/7
  Logical Operator1/1 -> Logical Operator8/2
  Logical Operator7/1 -> Logical Operator8/8
  Data_5(1b)/1 -> Logical Operator2/1
  Logical Operator8/1 -> Data(1b)/1
  Data_6(1b)/1 -> Logical Operator1/1
  Logical Operator10/1 -> Logical Operator4/3, Logical Operator5/3, Logical Operator7/3, Logical Operator6/3
  Addr_2(1b)/1 -> Logical Operator/3, Logical Operator1/3, Logical Operator3/3, Logical Operator2/3, Logical Operator10/1
  Logical Operator3/1 -> Logical Operator8/4
  Data_7(1b)/1 -> Logical Operator/1
  Logical Operator4/1 -> Logical Operator8/5
  Data_2(1b)/1 -> Logical Operator5/1
  Logical Operator5/1 -> Logical Operator8/6
  Data_0(1b)/1 -> Logical Operator7/1
  Data_1(1b)/1 -> Logical Operator6/1
